simulink model "project_external_resistive_load"  (R2015a)
settings: Solver=ode23tb  StartTime=0.0  StopTime=6000  RelTol=1e-4
undefined symbols (not defined in the file): Ion, Lithium
libraries: powerlib x10, electricdrivelib x1
settings Model: CovSFcnEnable=off  Creator=raj  LastModifiedBy=vaio

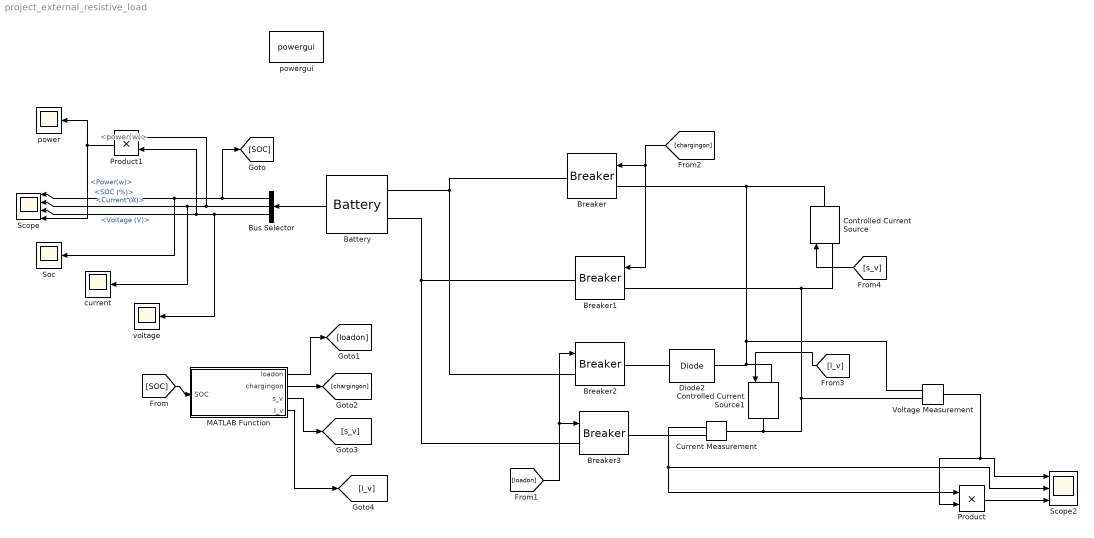
== system project_external_resistive_load ==
  note: <power(w)>
  Battery : electricdrivelib/Extra Sources/Battery  BatType=Lithium-Ion  ShowDetailedParameters=off  NomV=3.6  NomQ=2.25  SOC=13  PresetModel=on  MaxQ=2.25  FullV=4.1904  Dis_rate=0.97826  R=0.016  Normal_OP=2.0348  expZone="[3.8894     0.11054]"  current=[1.5 3]  Units=Ampere-hour  Batt_Tr=30
  Breaker : powerlib/Elements/Breaker  InitialState=0  SwitchingTimes="[1/60  5/60]"  External=on  BreakerResistance=0.01  SnubberResistance=1e6  SnubberCapacitance=inf  Measurements=Branch voltage and current  MoreParameters=on  NoBreakLoop=off
  Breaker1 : powerlib/Elements/Breaker  InitialState=0  SwitchingTimes="[1/60  5/60]"  External=on  BreakerResistance=0.01  SnubberResistance=1e6  SnubberCapacitance=inf  Measurements=None  MoreParameters=on  NoBreakLoop=off
  Breaker2 : powerlib/Elements/Breaker  InitialState=0  SwitchingTimes="[1/60  5/60]"  External=on  BreakerResistance=0.01  SnubberResistance=1e6  SnubberCapacitance=inf  Measurements=Branch voltage and current  MoreParameters=on  NoBreakLoop=off
  Breaker3 : powerlib/Elements/Breaker  InitialState=0  SwitchingTimes="[1/60  5/60]"  External=on  BreakerResistance=0.01  SnubberResistance=1e6  SnubberCapacitance=inf  Measurements=Branch voltage and current  MoreParameters=on  NoBreakLoop=off
  Bus Selector : BusSelector  OutputSignals=SOC (%),Current (A),Voltage (V)
  Controlled Current Source : powerlib/Electrical Sources/Controlled Current Source  Initialize=on  Source_Type=DC  Amplitude=1  Phase=0  Frequency=0  Measurements=Current
  Controlled Current Source1 : powerlib/Electrical Sources/Controlled Current Source  Initialize=on  Source_Type=DC  Amplitude=2  Phase=0  Frequency=0  Measurements=Current
  Current Measurement : powerlib/Measurements/Current Measurement  PhasorSimulation=off  OutputType=Complex  PSBequivalent=0
  Diode2 : powerlib/Power Electronics/Diode  Ron=0.0001  Lon=0  Vf=0.05  IC=0  UseSnubber=off  Rs=0  Cs=0  Measurements=off
  MATLAB Function : MATLAB Function  TreatAsAtomicUnit=on
  Product : Product
  Product1 : Product
  Scope : Scope  NumInputPorts=4
      settings: TimeRange=500  YMin=10~0.5~3.5~6.2  YMax=20~3~3.8~6.8  SaveName=soc
  Scope2 : Scope  NumInputPorts=3
      settings: YMin=-5~-5~-5  YMax=5~5~5  SaveName=ScopeData2
  "Soc " : Scope
      settings: SaveName=soc
  Voltage Measurement : powerlib/Measurements/Voltage Measurement  PhasorSimulation=off  OutputType=Complex  PSBequivalent=0
  current : Scope
      settings: SaveName=current
  "power " : Scope
      settings: SaveName=power
  powergui : powerlib/powergui  Priority=1  SimulationMode=Continuous  SolverType=Tustin  SampleTime=50e-6  frequency=60  SPID=off  DisableSnubberDevices=on  DisableRonSwitches=on  DisableVfSwitches=on  SwTol=0  DisplayEquations=on  Interpol=off  methode=off  Ts=100  FunctionMessages=off  echomessages=off  HookPort=off  EnableUseOfTLC=off  x0status=blocks  frequencyindice=0  Pbase=100e6  ErrMax=1e-4  Iterations=50  UnitsV=kV  UnitsW=MW  buscounter=0  RestoreLinks=warning  ResistiveCurrentMeasurement=off  Frange=[0:2:500]  Ylog=off  Xlog=on  ShowGrid=off  save=off  variable=ZData  structure=0  ZoomFFT=off  StartTime=0.0  cycles=1  DisplayStyle=1  fundamental=60  FreqAxis=off  MaxFrequency=1000  frequencyindicesteady=1  RmsSteady=1  display=off
  voltage : Scope
      settings: SaveName=voltage
  wires:
  Bus Selector/1 -> [SOC], "Soc "/1, Scope/1  "<SOC (%)>"
  Bus Selector/2 -> Product1/1, current/1, Scope/2  "<Current (A)>"
  Bus Selector/3 -> voltage/1, Product1/2, Scope/3  "<Voltage (V)>"
  Battery/1 -> Bus Selector/1
  Current Measurement/1 -> Scope2/2, Product/1
  Voltage Measurement/1 -> Product/2, Scope2/1
  Product/1 -> Scope2/3
  [SOC] -> MATLAB Function/1(SOC)
  MATLAB Function/2(chargingon) -> [chargingon]
  [loadon] -> Breaker3/1, Breaker2/1
  [chargingon] -> Breaker1/1, Breaker/1
  MATLAB Function/3(s_v) -> [s_v]
  MATLAB Function/1(loadon) -> [loadon]
  Product1/1 -> Scope/4, "power "/1  "<Power(w)>"
  [s_v] -> Controlled Current Source/1
  [l_v] -> Controlled Current Source1/1
  MATLAB Function/4(l_v) -> [l_v]
  connections:
  Breaker2/LConn1 -- Breaker/RConn1 -- Battery/LConn1
  Breaker3/LConn1 -- Breaker1/RConn1 -- Battery/LConn2
  Current Measurement/RConn1 -- Breaker3/RConn1
  Diode2/LConn1 -- Breaker2/RConn1
  Controlled Current Source/RConn1 -- Voltage Measurement/LConn1 -- Controlled Current Source1/LConn1 -- Diode2/RConn1 -- Breaker/LConn1
  Controlled Current Source/LConn1 -- Voltage Measurement/LConn2 -- Controlled Current Source1/RConn1 -- Current Measurement/LConn1 -- Breaker1/LConn1

== matlab function project_external_resistive_load/MATLAB Function ==
  data: SOC input; loadon output; chargingon output; s_v output; l_v output
function[loadon,chargingon,s_v,l_v]=fcn(SOC)
loadon=1;
chargingon=0;
s_v=0.23;%5
l_v=2;

if(SOC>=90)

    loadon=1;
    chargingon=0;
    s_v=0.23;%5
    l_v=2;
    
end
if(SOC<=10)

    loadon=0;
    chargingon=1;
    s_v=5;%5
    l_v=2;
 
end

end
